simulink model "Lab2_PartA3"  (R2025b)
settings: Solver=VariableStepAuto  StartTime=0.0  StopTime=10.0  RelTol=1e-3
libraries: SignalEditorBlockLib x2
settings Model: Creator=Murl0  LastModifiedBy=Murl0

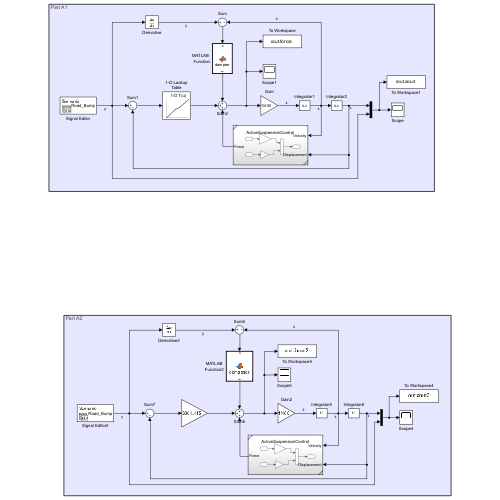
[thumbnail: Simulink's stored preview of the top-level diagram]
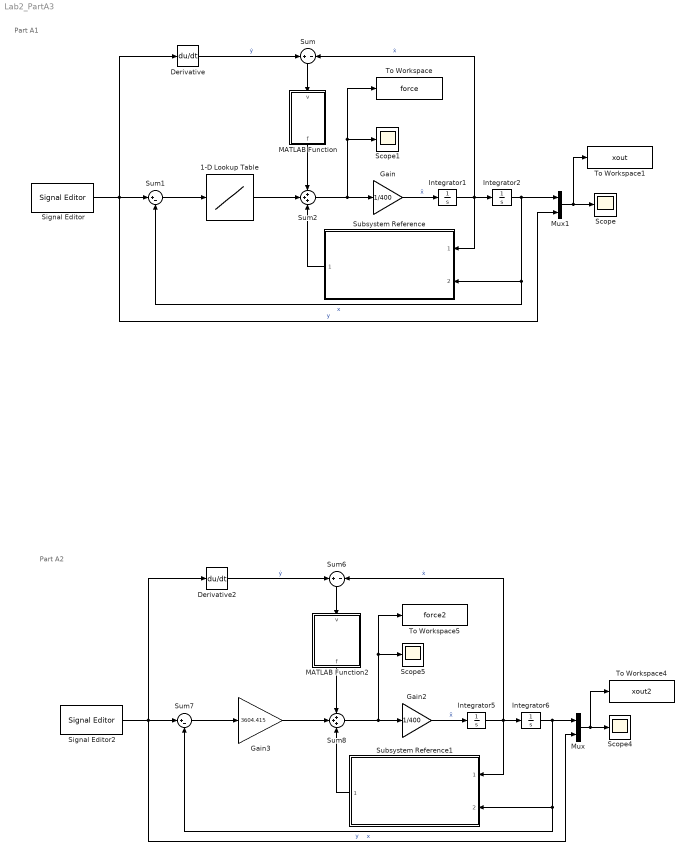
== system Lab2_PartA3 ==
  note: Part A1
  note: Part A2
  1-D Lookup Table : Lookup_n-D  NumberOfTableDimensions=1  BreakpointsForDimension1=[-0.5;-0.1;0;0.1;0.5]  Table=[-4500;-500;0;500;4500]  InternalRulePriority=Speed  RndMeth=Simplest
  Derivative : Derivative
  Derivative2 : Derivative
  Gain : Gain  Gain=1/400
  Gain2 : Gain  Gain=1/400
  Gain3 : Gain  Gain=3604.415
  Integrator{1..2,5..6} (4 alike) : Integrator
  MATLAB Function : MATLAB Function  TreatAsAtomicUnit=on
  MATLAB Function2 : MATLAB Function  TreatAsAtomicUnit=on
  Mux : Mux  Inputs=2
  Mux1 : Mux  Inputs=2
  Scope{,1,4..5} (4 alike) : Scope
      Scope settings: ActiveDisplayYMinimum=-1.4940400064433929E+11  ActiveDisplayYMaximum=1.6675311941656321E+10
      Scope1 settings: ActiveDisplayYMinimum=-3855.4098186727856  ActiveDisplayYMaximum=-0.63420787282950641
      Scope4 settings: ActiveDisplayYMinimum=-0.024999999999999994  ActiveDisplayYMaximum=0.225  DataLoggingVariableName=ScopeData4
      Scope5 settings: ActiveDisplayYMinimum=-0.034259677699392782  ActiveDisplayYMaximum=0.22642326638111926  DataLoggingVariableName=ScopeData5
  Signal Editor : SignalEditorBlockLib/Signal Editor  FileName=Input.mat  ActiveScenario=Scenario  ActiveSignal=Road_Bump  IsBus=off  OutputBusObjectStr=Bus: BusObject  SampleTime=0  ZeroCross=off  OutputAfterFinalValue=Setting to zero  Unit=m  PreserveSignalName=on  ApplySigPropsToAllScenarios=on  ApplySigPropsToAllSignals=off  SignalPropertySource=Dialog parameters
  Signal Editor2 : SignalEditorBlockLib/Signal Editor  FileName=Input.mat  ActiveScenario=Scenario  ActiveSignal=Road_Bump  IsBus=off  OutputBusObjectStr=Bus: BusObject  SampleTime=0  ZeroCross=off  OutputAfterFinalValue=Setting to zero  Unit=m  PreserveSignalName=on  ApplySigPropsToAllScenarios=on  ApplySigPropsToAllSignals=off  SignalPropertySource=Dialog parameters
  Subsystem Reference : Subsystem  ReferencedSubsystem=ActiveSuspensionControl
  Subsystem Reference1 : Subsystem  ReferencedSubsystem=ActiveSuspensionControl
  Sum : Sum  Inputs=+-
  Sum1 : Sum  Inputs=|+-
  Sum2 : Sum  Inputs=+++
  Sum6 : Sum  Inputs=+-
  Sum7 : Sum  Inputs=|+-
  Sum8 : Sum  Inputs=+++
  To Workspace : ToWorkspace  VariableName=force  SampleTime=-1
  To Workspace1 : ToWorkspace  VariableName=xout  SampleTime=-1
  To Workspace4 : ToWorkspace  VariableName=xout2  SampleTime=-1
  To Workspace5 : ToWorkspace  VariableName=force2  SampleTime=-1
  wires:
  Integrator2/1 -> Mux1/1, Sum1/2, Subsystem Reference/2  "x"
  Integrator1/1 -> Subsystem Reference/1, Sum/2, Integrator2/1  "ẋ"
  Gain/1 -> Integrator1/1  "ẍ"
  Sum2/1 -> Gain/1, Scope1/1, To Workspace/1
  MATLAB Function/1(f) -> Sum2/1
  Sum/1 -> MATLAB Function/1(v)
  Derivative/1 -> Sum/1  "ẏ"
  1-D Lookup Table/1 -> Sum2/2
  Sum1/1 -> 1-D Lookup Table/1
  Signal Editor/1 -> Mux1/2, Sum1/1, Derivative/1  "y"
  Subsystem Reference/1 -> Sum2/3
  MATLAB Function2/1(f) -> Sum8/1
  Sum7/1 -> Gain3/1
  Integrator6/1 -> Mux/1, Sum7/2, Subsystem Reference1/2  "x"
  Gain2/1 -> Integrator5/1  "ẍ"
  Gain3/1 -> Sum8/2
  Integrator5/1 -> Subsystem Reference1/1, Sum6/2, Integrator6/1  "ẋ"
  Sum6/1 -> MATLAB Function2/1(v)
  Derivative2/1 -> Sum6/1  "ẏ"
  Signal Editor2/1 -> Mux/2, Derivative2/1, Sum7/1  "y"
  Subsystem Reference1/1 -> Sum8/3
  Mux1/1 -> To Workspace1/1, Scope/1
  Mux/1 -> Scope4/1, To Workspace4/1
  Sum8/1 -> Gain2/1, Scope5/1, To Workspace5/1

== matlab function Lab2_PartA3/MATLAB Function2 ==
  data: f output; v input
function f = dampener(v)
% Linear damper model
% Input: v = (ydot - xdot)
% Output: f = b * (ydot - xdot)

b = 84.056;   % Damping coefficient (N·s/m)
f = b * v;    % Linear damping force
end

== matlab function Lab2_PartA3/MATLAB Function ==
  data: v input; f output
function f = damper(v)

if v<= 0
    f = -800*(abs(v)).^(0.6);
else
    f = 200*v.^(0.6);
end
